simulink model "zad1"  (R2020b)
settings: Solver=FixedStepDiscrete  StartTime=0.0  StopTime=0.0  RelTol=1e-3
libraries: CPOiS_SourcesSinks x7, CPOiS_DataManipulation x4, CPOiS_DataManipulation_IntroduceNoise x2, CPOiS_Filters x2, CPOiS_General x1
settings Model: Creator=jrybarz  LastModifiedBy=jrybarz

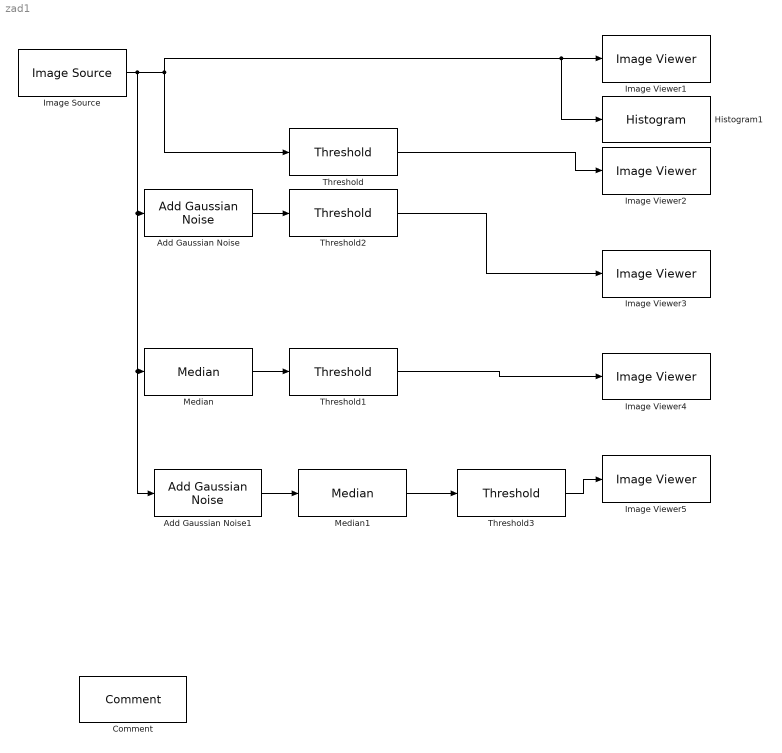
== system zad1 ==
  Add Gaussian Noise : CPOiS_DataManipulation_IntroduceNoise/Add Gaussian Noise  Mean=0  Variance=10.0
      settings: SourceProductName=CPOiS - Digital image and signal processing
  Add Gaussian Noise1 : CPOiS_DataManipulation_IntroduceNoise/Add Gaussian Noise  Mean=0  Variance=10.0
      settings: SourceProductName=CPOiS - Digital image and signal processing
  Comment : CPOiS_General/Comment
      settings: SourceProductName=CPOiS - Digital image and signal processing
  Histogram1 : CPOiS_SourcesSinks/Histogram
      settings: SourceProductName=CPOiS - Digital image and signal processing
  Image Source : CPOiS_SourcesSinks/Image Source  FileSelection=gull.png
      settings: SourceProductName=CPOiS - Digital image and signal processing
  Image Viewer{1..5} (5 alike) : CPOiS_SourcesSinks/Image Viewer
      settings: SourceProductName=CPOiS - Digital image and signal processing
  Median : CPOiS_Filters/Median  MaskSize=3 x 3
      settings: SourceProductName=CPOiS - Digital image and signal processing
  Median1 : CPOiS_Filters/Median  MaskSize=3 x 3
      settings: SourceProductName=CPOiS - Digital image and signal processing
  Threshold{,1..3} (4 alike) : CPOiS_DataManipulation/Threshold  Threshold=127
      settings: SourceProductName=CPOiS - Digital image and signal processing
  wires:
  Image Source/1 -> Add Gaussian Noise1/1, Median/1, Add Gaussian Noise/1, Threshold/1, Histogram1/1, Image Viewer1/1
  Add Gaussian Noise/1 -> Threshold2/1
  Threshold/1 -> Image Viewer2/1
  Threshold2/1 -> Image Viewer3/1
  Add Gaussian Noise1/1 -> Median1/1
  Median/1 -> Threshold1/1
  Median1/1 -> Threshold3/1
  Threshold1/1 -> Image Viewer4/1
  Threshold3/1 -> Image Viewer5/1
